simulink model "Schnittstelle_mit_Gewerk1"  (R2015b)
settings: Solver=VariableStepAuto  StartTime=0.0  StopTime=10.0  RelTol=1e-3
settings Model: Creator=atlabor  LastModifiedBy=atlabor

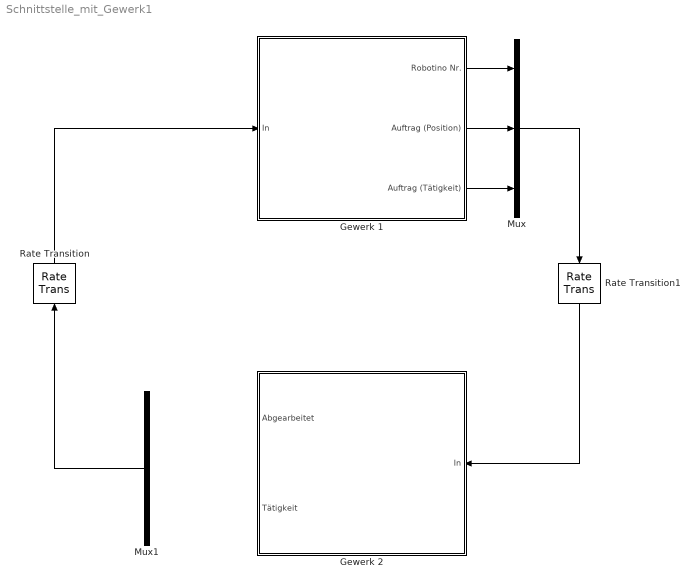
== system Schnittstelle_mit_Gewerk1 ==
  Gewerk 1 : Subsystem
  Gewerk 2 : Subsystem
  Mux : Mux  Inputs=3
  Mux1 : Mux  Inputs=3
  Rate Transition : RateTransition
  Rate Transition1 : RateTransition
  wires:
  Rate Transition/1 -> Gewerk 1/1(In)
  Rate Transition1/1 -> Gewerk 2/1(In)
  Mux/1 -> Rate Transition1/1
  Mux1/1 -> Rate Transition/1
  Gewerk 1/3(Auftrag (Tätigkeit)) -> Mux/3
  Gewerk 1/2(Auftrag (Position)) -> Mux/2
  Gewerk 1/1(Robotino Nr.) -> Mux/1

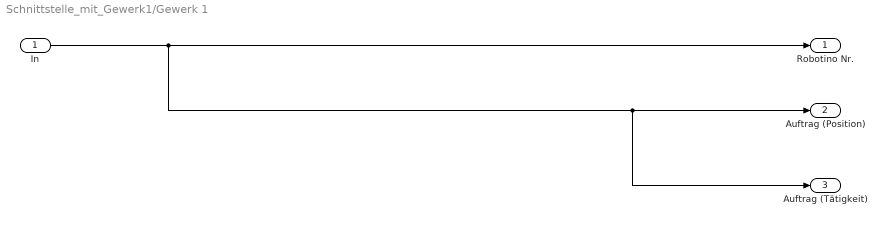
== system Schnittstelle_mit_Gewerk1/Gewerk 1 ==
  In : Inport
  Robotino Nr. : Outport
  Auftrag (Position) : Outport  Port=2
  Auftrag (Tätigkeit) : Outport  Port=3
  wires:
  In/1 -> Auftrag (Tätigkeit)/1, Auftrag (Position)/1, Robotino Nr./1

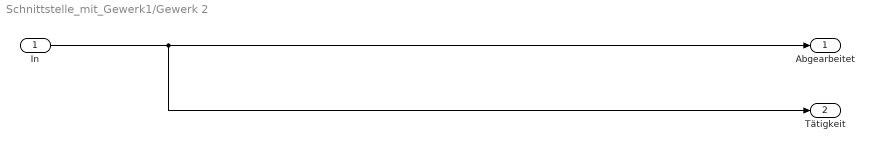
== system Schnittstelle_mit_Gewerk1/Gewerk 2 ==
  In : Inport
  Abgearbeitet : Outport
  Tätigkeit : Outport  Port=2
  wires:
  In/1 -> Abgearbeitet/1, Tätigkeit/1
